simulink model "Exp"  (R2017b)
settings: Solver=FixedStepAuto  StartTime=0.0  StopTime=inf  FixedStep=ts  RelTol=1e-3  EnableMultiTasking=on
values from neighbouring files (symbols this model uses):
  acc_gain = 50    [Init_Exp.m]
  cc = 16    [Init_Exp.m]
  channel = 5    [Init_Exp.m]
  f_gait = 0.1    [Init_Exp.m]
  Kg = 80    [Init_Exp.m]
  R_k = diag([1E-4*[1;1];1E-6*[1;1]])    [Init_Exp.m]
  sigma_p = [0.5 1 100000 100000 100000 100000]'    [Init_Exp.m]
  sigma_pp = [sigma sigma sigma sigma sigma sigma]'    [Init_Exp.m]
  sigma_r = [100000 100000 100000 100000]'    [Init_Exp.m]
  sigma_rr = [sigma sigma sigma sigma]'    [Init_Exp.m]
  systemP = [tau_c2,tau_s2,dqs2,eta2,X2,Y2,J2,tau_c1,tau_s1,dqs1,eta1,X1,Y1,J1]    [Init_Exp.m]
  ts = 0.001    [Init_Exp.m]
  vard = vardtimes*1E-2*[2;1]    [Init_Exp.m]
  vardq = 1E-4*[1;1]    [Init_Exp.m]
  varq = 1E-5*[1;1]    [Init_Exp.m]
undefined symbols (not defined in the file or in its folder): acceleration, command, cxk, desired_acc, desired_position, desired_velocity, DiscIntNeverNeededParam, disturbance, immxk, interaction_force, mkxk, motor_torque, observer, position, velocity, xk
libraries: xpcethercatlib x37, slrtlib x9, simulink x1
(part 2 of 2)

== matlab function Exp/Control/Feedforward&nonlinearFeekbackLinearlization&Observer/disturbance observer ==
  data: TT output; q input; dq input; ddq input; cur input; para input; z input; zz output; d output; c input
function [TT,zz,d] = fcn(q,dq,ddq,cur,para,z,c)


l1=0.42;
tau_c2=para(1);
tau_s2=para(2);
dqs2=para(3);
eta2=para(4);
X2=para(5);
Y2=para(6);
J2=para(7);

tau_c1=para(8);
tau_s1=para(9);
dqs1=para(10);
eta1=para(11);
X1=para(12);
Y1=para(13);
J1=para(14);




%% M matrix
M11=J1+2*l1*(X2*cos(q(2))-Y2*sin(q(2)));
M12=J2+l1*(X2*cos(q(2))-Y2*sin(q(2)));
M21=J2+l1*(X2*cos(q(2))-Y2*sin(q(2)));
M22=J2;

M=[M11,M12;M21,M22];
%% C matrix
C11=-2*l1*(X2*sin(q(2))+Y2*cos(q(2))).*dq(2);
C12=-l1*(X2*sin(q(2))+Y2*cos(q(2))).*dq(2);
C21=l1*(X2*sin(q(2))+Y2*cos(q(2))).*dq(1);
C22=0;

C=[C11,C12;C21,C22];
%% G matrix
G1=9.7925*(X1*sin(q(1))+Y1*cos(q(1)+X2*sin(q(1)+q(2))+Y2*cos(q(1)+q(2))));
G2=9.7925*(X2*sin(q(1)+q(2))+Y2*cos(q(1)+q(2)));

G=[G1;G2];

%% F matrix
F1=(tau_c1+(tau_s1-tau_c1)*exp(-dq(1)/dqs1)).*customSIGN(dq(1))+eta1*dq(1);
F2=(tau_c2+(tau_s2-tau_c2)*exp(-dq(2)/dqs2)).*customSIGN(dq(2))+eta2*dq(2);


F=[F1;F2];

%%

TT=M*ddq+C*dq+G+F;

%% obtain T
% T=cur-F;
T=cur;

%% nonlinear disturbance observer

p=c*[dq(1),dq(1)+dq(2)]';


dt=0.001;
% obtain L matrix
L=c*[1,0;1,1]/M;
zz=(eye(2)-L*dt)*z+L*dt*(C*dq+G-T-p);

d=zz+p;





end



function y=customSIGN(u)
threshold=0.05;
if(u>threshold)
    y=1;
elseif(u<-threshold)
    y=-1;
else
    y=u/threshold;
end


end

== matlab function Exp/Control/Feedforward&nonlinearFeekbackLinearlization&Observer/extended kalman filter ==
  data: xkk output; d output; q input; dq input; ddq input; cur input; para input; D output; xk input; Q_k input; R_k input
function [xkk,d, D] = ExtendedKalmanFilter(q,dq,ddq,cur,para,xk,Q_k,R_k)


persistent   Pk;

if isempty(Pk)
    Pk= 10*eye(6);
end

dt=0.001;
l1=0.42;
tau_c2=para(1);
tau_s2=para(2);
dqs2=para(3);
eta2=para(4);
X2=para(5);
Y2=para(6);
J2=para(7);
tau_c1=para(8);
tau_s1=para(9);
dqs1=para(10);
eta1=para(11);
X1=para(12);
Y1=para(13);
J1=para(14);
%% M matrix
M11=J1+2*l1*(X2*cos(q(2))-Y2*sin(q(2)));
M12=J2+l1*(X2*cos(q(2))-Y2*sin(q(2)));
M21=J2+l1*(X2*cos(q(2))-Y2*sin(q(2)));
M22=J2;
M=[M11,M12;M21,M22];
%% C matrix
C11=-2*l1*(X2*sin(q(2))+Y2*cos(q(2))).*dq(2);
C12=-l1*(X2*sin(q(2))+Y2*cos(q(2))).*dq(2);
C21=l1*(X2*sin(q(2))+Y2*cos(q(2))).*dq(1);
C22=0;
C=[C11,C12;C21,C22];
%% G matrix
G1=9.7925*(X1*sin(q(1))+Y1*cos(q(1)+X2*sin(q(1)+q(2))+Y2*cos(q(1)+q(2))));
G2=9.7925*(X2*sin(q(1)+q(2))+Y2*cos(q(1)+q(2)));
G=[G1;G2];
%% F matrix：fraction
F1=(tau_c1+(tau_s1-tau_c1)*exp(-dq(1)/dqs1)).*customSIGN(dq(1))+eta1*dq(1);
F2=(tau_c2+(tau_s2-tau_c2)*exp(-dq(2)/dqs2)).*customSIGN(dq(2))+eta2*dq(2);
F=[F1;F2];
F=[0;0];
%% native disturbance
D= -cur + (M*ddq+C*dq+G+F);

%% Extended Kalman filter
    H_k = [ 0,0,1,0,0,0;0,0,0,1,0,0;0,0,0,0,1,0;0,0,0,0,0,1];

    y_k = [dq(1),dq(2),q(1),q(2)]';
    % obtain fx
    xdotk=getfxk_1(xk, cur,M,C,G, F);
    xk_=xk + xdotk *dt ;
    
    % obtain F_k
    F_k = GetJacobian_1(xk , cur, F,para);
    
    Pk_=F_k * Pk *  F_k' + Q_k ;
    
    K_k = Pk_ * H_k' /(H_k * Pk_ * H_k' + R_k); 
    
    % Pk = (eye(6)- K_k * H_k)*Pk_;
    Pk = (eye(6)- K_k * H_k)*Pk_*(eye(6)- K_k * H_k)'+ K_k* R_k*K_k';
    
    xkk= xk_ + K_k*(y_k - H_k*xk_);
    
    d =[xkk(1),xkk(2)]';
    
end

function xdot=getfxk_1(x, T, M, C, G, F)

% x= [d dq q]
d=x(1:2);
dq=x(3:4);
q=x(5:6);
invM=inv(M);

xdot=zeros(6,1);
xdot(1:2)=zeros(2,1);
xdot(3:4)=invM*(T+d-C*dq-G-F);

xdot(5:6)=dq;

end

function F_k = GetJacobian_1(x, T, F, para)


dt=0.001;
l1=0.42;
g=9.7925;
X2=para(5);
Y2=para(6);
J2=para(7);
X1=para(12);
Y1=para(13);
J1=para(14);

d=x(1:2);
dq=x(3:4);
q=x(5:6);
%% M matrix
M11=J1+2*l1*(X2*cos(q(2))-Y2*sin(q(2)));
M12=J2+l1*(X2*cos(q(2))-Y2*sin(q(2)));
M21=J2+l1*(X2*cos(q(2))-Y2*sin(q(2)));
M22=J2;
M=[M11,M12;M21,M22];
%% C matrix
C11=-2*l1*(X2*sin(q(2))+Y2*cos(q(2))).*dq(2);
C12=-l1*(X2*sin(q(2))+Y2*cos(q(2))).*dq(2);
C21=l1*(X2*sin(q(2))+Y2*cos(q(2))).*dq(1);
C22=0;
C=[C11,C12;C21,C22];
%% G matrix
G1=g*(X1*sin(q(1))+Y1*cos(q(1)+X2*sin(q(1)+q(2))+Y2*cos(q(1)+q(2))));
G2=g*(X2*sin(q(1)+q(2))+Y2*cos(q(1)+q(2)));
G=[G1;G2];
invM=inv(M);
% calculate xdot
xdot=zeros(6,1);
xdot(1:2)=zeros(2,1);
xdot(3:4)=invM*(T+d-C*dq-G-F);
xdot(5:6)=dq;

f_xk =  xdot;
%%  obtain the numerical Jacobian matrix
gra = zeros(6,6);
for i=1:6
scale = 1E-6;
delta=zeros(6,1);
delta(i)=scale;
%% calculate x_del
x_del=x + delta;
d_del=x_del(1:2);
dq_del=x_del(3:4);
q_del=x_del(5:6);
%% M matrix
M11=J1+2*l1*(X2*cos(q_del(2))-Y2*sin(q_del(2)));
M12=J2+l1*(X2*cos(q_del(2))-Y2*sin(q_del(2)));
M21=J2+l1*(X2*cos(q_del(2))-Y2*sin(q_del(2)));
M22=J2;
M_del=[M11,M12;M21,M22];
%% C matrix
C11=-2*l1*(X2*sin(q_del(2))+Y2*cos(q_del(2))).*dq_del(2);
C12=-l1*(X2*sin(q_del(2))+Y2*cos(q_del(2))).*dq_del(2);
C21=l1*(X2*sin(q_del(2))+Y2*cos(q_del(2))).*dq_del(1);
C22=0;
C_del=[C11,C12;C21,C22];
%% G matrix
G1=g*(X1*sin(q_del(1))+Y1*cos(q_del(1)+X2*sin(q_del(1)+q_del(2))+Y2*cos(q_del(1)+q_del(2))));
G2=g*(X2*sin(q_del(1)+q_del(2))+Y2*cos(q_del(1)+q_del(2)));
G_del=[G1;G2];
invM_del=inv(M_del);
% calculate xdot_del
xdot_del=zeros(6,1);
xdot_del(1:2)=zeros(2,1);
xdot_del(3:4)=invM_del*(T+d_del-C_del*dq_del-G_del-F);
xdot_del(5:6)=dq_del;

f_xk_del= xdot_del ;

J_delta=(f_xk_del - f_xk)*dt;
gra(i,:)=J_delta/scale;

end

F_k = gra'+ eye(6);

end

function y=customSIGN(u)
threshold=0.05;
if(u>threshold)
    y=1;
elseif(u<-threshold)
    y=-1;
else
    y=u/threshold;
end

end

== matlab function Exp/Emergency/MATLAB Function ==
  data: position input; y output; force input
function y = fcn(position, force)

y=0;

if position(1)>0.25*2*pi||position(1)<-0.25*2*pi...
        ||position(2)>0.25*2*pi||position(2)<-0.28*2*pi...
        ||position(3)>0.25*2*pi||position(3)<-0.25*2*pi...
        ||position(4)>0.25*2*pi||position(4)<-0.28*2*pi
    y=1;
else
    y=y;
end

== matlab function Exp/Control/Feedforward&nonlinearFeekbackLinearlization&Observer/MKEKF ==
  data: xkk output; d output; q input; dq input; ddq input; cur input; para input; D output; xk input; num output; Q_k input; Q_maxk input; R_k input; sigma_p input; sigma_r input; XE output; Pk1 output; vec_recp output
function [xkk,d, D,num,XE,Pk1,vec_recp] = MltiKernelExtendedKalmanFilter(q,dq,ddq,cur,para,xk,Q_k,Q_maxk,R_k,sigma_p,sigma_r)


persistent  Pk;

if isempty(Pk)
    Pk= 0.001*eye(6);
end

dt=0.001;
l1=0.42;
tau_c2=para(1);
tau_s2=para(2);
dqs2=para(3);
eta2=para(4);
X2=para(5);
Y2=para(6);
J2=para(7);
tau_c1=para(8);
tau_s1=para(9);
dqs1=para(10);
eta1=para(11);
X1=para(12);
Y1=para(13);
J1=para(14);
%% M matrix
M11=J1+2*l1*(X2*cos(q(2))-Y2*sin(q(2)));
M12=J2+l1*(X2*cos(q(2))-Y2*sin(q(2)));
M21=J2+l1*(X2*cos(q(2))-Y2*sin(q(2)));
M22=J2;
M=[M11,M12;M21,M22];
%% C matrix
C11=-2*l1*(X2*sin(q(2))+Y2*cos(q(2))).*dq(2);
C12=-l1*(X2*sin(q(2))+Y2*cos(q(2))).*dq(2);
C21=l1*(X2*sin(q(2))+Y2*cos(q(2))).*dq(1);
C22=0;
C=[C11,C12;C21,C22];
%% G matrix
G1=9.7925*(X1*sin(q(1))+Y1*cos(q(1)+X2*sin(q(1)+q(2))+Y2*cos(q(1)+q(2))));
G2=9.7925*(X2*sin(q(1)+q(2))+Y2*cos(q(1)+q(2)));
G=[G1;G2];
%% F matrix
F1=(tau_c1+(tau_s1-tau_c1)*exp(-dq(1)/dqs1)).*customSIGN(dq(1))+eta1*dq(1);
F2=(tau_c2+(tau_s2-tau_c2)*exp(-dq(2)/dqs2)).*customSIGN(dq(2))+eta2*dq(2);
F=[F1;F2];
F=[0;0];
%% native disturbance
D= -cur + (M*ddq+C*dq+G+F);

%% Extended Kalman filter
%     sigma_p=[0.5 2 100000 100000 100000 100000]';
%     sigma_r=[100000 100000 100000 100000]';
    H_k = [ 0,0,1,0,0,0;0,0,0,1,0,0;0,0,0,0,1,0;0,0,0,0,0,1];

    y_k = [dq(1),dq(2),q(1),q(2)]';
    % obtain fx
    xdotk=getfxk_1(xk, cur,M,C,G, F);
    xk_=xk + xdotk *dt ;
    
    % obtain F_k
    F_k = GetJacobian_1(xk , cur, F,para);
    
   Pk_=F_k * Pk *  F_k' + Q_k ;   
   %% 
   Pk_max=F_k * Pk *  F_k' + Q_maxk;
   vec_amp=diag(Pk_max)./diag(Pk_);
   vec_recp=1./vec_amp;
   %% %% mkekf
    num=3;
    cnt=num;
    X_t=zeros(6,1);
    K_1=zeros(6,4);
    P_1=zeros(6,6);
    R_1=zeros(4,4);
    XE=zeros(cnt,1);
    %bp = chol(Pk_,'lower') ;
    %Pk_p1=diag(diag(Pk_));
    %Pk_p2=Pk_-Pk_p1;
    bp = chol(Pk_,'lower') ;
    %bp = chol(Pk_p1,'lower') ;
    br = chol(R_k,'lower') ;
    while(num>0) 
    dp= bp\xk_;
    dr= br\y_k;
        % 
    if(num==cnt)
      X_tlast=xk_; 
    else  
      X_tlast=X_t; 
    end
    wp= bp\X_tlast;
    wr= (br)\H_k*X_tlast;
    ep=dp-wp;
    er=dr-wr;
    %  P_ and R
    Cx_array=exp(-ep.*ep./(2*sigma_p.*sigma_p));
    Cy_array=exp(-er.*er./(2*sigma_r.*sigma_r));
    for kk=1:6
        if(Cx_array(kk)<vec_recp(kk))
            Cx_array(kk)=vec_recp(kk);
            num=1;
        end
    end
    
    
    Cx=diag(Cx_array);
    Cy=diag(Cy_array);
        
    R_1=br/Cy*br';
    P_1=bp/Cx*bp';
    %P_1=bp/Cx*bp'+Pk_p2;
    K_1=P_1*H_k'/(H_k*P_1*H_k'+R_1);  
    X_t=xk_+K_1*(y_k-H_k*xk_); 
    
    num=num-1;    
    xe=norm(X_t-X_tlast)/(norm(X_tlast)+0.00001);
    XE(cnt-num)=xe;
    if(xe<0.005)
        break
    end
    
    end 
    %%%%
   
    Pk = (eye(6)- K_1 * H_k)*P_1*(eye(6)- K_1 * H_k)'+ K_1* R_1*K_1';
        
    xkk= X_t;
    
    d =[xkk(1),xkk(2)]';
    
    Pk1=diag(Pk);
end

function xdot=getfxk_1(x, T, M, C, G, F)

% x= [d dq q]
d=x(1:2);
dq=x(3:4);
q=x(5:6);
invM=inv(M);

xdot=zeros(6,1);
xdot(1:2)=zeros(2,1);
xdot(3:4)=invM*(T+d-C*dq-G-F);
xdot(5:6)=dq;

end
function F_k = GetJacobian_1(x, T, F, para)


dt=0.001;
l1=0.42;
g=9.7925;
X2=para(5);
Y2=para(6);
J2=para(7);
X1=para(12);
Y1=para(13);
J1=para(14);

d=x(1:2);
dq=x(3:4);
q=x(5:6);
%% M matrix
M11=J1+2*l1*(X2*cos(q(2))-Y2*sin(q(2)));
M12=J2+l1*(X2*cos(q(2))-Y2*sin(q(2)));
M21=J2+l1*(X2*cos(q(2))-Y2*sin(q(2)));
M22=J2;
M=[M11,M12;M21,M22];
%% C matrix
C11=-2*l1*(X2*sin(q(2))+Y2*cos(q(2))).*dq(2);
C12=-l1*(X2*sin(q(2))+Y2*cos(q(2))).*dq(2);
C21=l1*(X2*sin(q(2))+Y2*cos(q(2))).*dq(1);
C22=0;
C=[C11,C12;C21,C22];
%% G matrix
G1=g*(X1*sin(q(1))+Y1*cos(q(1)+X2*sin(q(1)+q(2))+Y2*cos(q(1)+q(2))));
G2=g*(X2*sin(q(1)+q(2))+Y2*cos(q(1)+q(2)));
G=[G1;G2];
invM=inv(M);
% calculate xdot
xdot=zeros(6,1);
xdot(1:2)=zeros(2,1);
xdot(3:4)=invM*(T+d-C*dq-G-F);
xdot(5:6)=dq;

f_xk =  xdot;
%%  obtain the numerical Jacobian matrix
gra = zeros(6,6);
for i=1:6
scale = 1E-4;
delta=zeros(6,1);
delta(i)=scale;
%% calculate x_del
x_del=x + delta;
d_del=x_del(1:2);
dq_del=x_del(3:4);
q_del=x_del(5:6);
%% M matrix
M11=J1+2*l1*(X2*cos(q_del(2))-Y2*sin(q_del(2)));
M12=J2+l1*(X2*cos(q_del(2))-Y2*sin(q_del(2)));
M21=J2+l1*(X2*cos(q_del(2))-Y2*sin(q_del(2)));
M22=J2;
M_del=[M11,M12;M21,M22];
%% C matrix
C11=-2*l1*(X2*sin(q_del(2))+Y2*cos(q_del(2))).*dq_del(2);
C12=-l1*(X2*sin(q_del(2))+Y2*cos(q_del(2))).*dq_del(2);
C21=l1*(X2*sin(q_del(2))+Y2*cos(q_del(2))).*dq_del(1);
C22=0;
C_del=[C11,C12;C21,C22];
%% G matrix
G1=g*(X1*sin(q_del(1))+Y1*cos(q_del(1)+X2*sin(q_del(1)+q_del(2))+Y2*cos(q_del(1)+q_del(2))));
G2=g*(X2*sin(q_del(1)+q_del(2))+Y2*cos(q_del(1)+q_del(2)));
G_del=[G1;G2];
invM_del=inv(M_del);
% calculate xdot_del
xdot_del=zeros(6,1);
xdot_del(1:2)=zeros(2,1);
xdot_del(3:4)=invM_del*(T+d_del-C_del*dq_del-G_del-F);
xdot_del(5:6)=dq_del;

f_xk_del= xdot_del ;

J_delta=(f_xk_del - f_xk)*dt;
gra(i,:)=J_delta/scale;

end

F_k = gra'+ eye(6);

end

function y=customSIGN(u)
threshold=0.05;
if(u>threshold)
    y=1;
elseif(u<-threshold)
    y=-1;
else
    y=u/threshold;
end

end

== matlab function Exp/6 Axis Force//Torque Sensor/MATLAB Function ==
  data: time input; Bias input; y input; y output; Bias output
function [y, Bias] = fcn(time, Bias, y)

if time <= 3 
    Bias=y;
    y=y*0;
else
    y=y-Bias;
end

end

== matlab function Exp/Control/Feedforward&nonlinearFeekbackLinearlization&Observer/process  ==
  data: vard input; Q_k output; vardq input; varq input
function Q_k = fcn(vard,vardq,varq)

Q_k= diag([vard;vardq;varq]);

== matlab function Exp/Control/Feedforward&nonlinearFeekbackLinearlization&Observer/process 1 ==
  data: vard input; Q_k output; vardq input; varq input; Q_maxk output
function [Q_k,Q_maxk] = fcn(vard,vardq,varq)

Q_k= diag([vard;vardq;varq]);

vardmax=20*1E-2*[2;1];
Q_maxk= diag([vardmax;vardq;varq]);

== matlab function Exp/Control/PD controller/MATLAB Function ==
  data: vele input; y output
function y = fcn(vele)

persistent  veleArr;

if isempty(veleArr)
    veleArr= zeros(20,2);
end

veleArr=circshift(veleArr,1);
veleArr(1,:)=vele;
y1 = var(veleArr(:,1));
y2 = var(veleArr(:,2));
y=[y1;y2];

== matlab function Exp/Emergency/MATLAB Function1 ==
  data: velvar input; y output
function y = fcn(velvar)

if(velvar(1)>0.04||velvar(2)>0.04)
    y=1;
else
    y=0;
end

end

== matlab function Exp/Emergency/MATLAB Function2 ==
  data: cmd input; y output
function y = fcn(cmd)

if(cmd(3)>80||cmd(4)>80)
    y=1;
else
    y=0;
end

end

== matlab function Exp/Control/Feedforward&nonlinearFeekbackLinearlization&Observer/extended kalman filter1 ==
  data: xkk output; xkk1 output; xkk2 output; d output; q input; dq input; cur input; para input; GAMMA output; Qk1 input; Qk2 input; Rk input; T input; mu output; Pkdiag output
function [xkk,xkk1,xkk2,d, GAMMA,mu,Pkdiag] = ExtendedKalmanFilterIMM(q,dq,cur,para,Qk1,Qk2,Rk,T)


persistent  Pk1 Pk2 x1 x2 mu1 mu2

if isempty(Pk1)
    Pk1= 1*eye(6);
end
if isempty(Pk2)
    Pk2= 1*eye(6);
end
if isempty(x1)
    x1= zeros(6,1)+0.01*ones(6,1);
end
if isempty(x2)
    x2= zeros(6,1);
end
if isempty(mu1)
    mu1= 0.5;
end
if isempty(mu2)
    mu2= 0.5;
end

dt=0.001;
l1=0.42;
tau_c2=para(1);
tau_s2=para(2);
dqs2=para(3);
eta2=para(4);
X2=para(5);
Y2=para(6);
J2=para(7);
tau_c1=para(8);
tau_s1=para(9);
dqs1=para(10);
eta1=para(11);
X1=para(12);
Y1=para(13);
J1=para(14);
%% M matrix
M11=J1+2*l1*(X2*cos(q(2))-Y2*sin(q(2)));
M12=J2+l1*(X2*cos(q(2))-Y2*sin(q(2)));
M21=J2+l1*(X2*cos(q(2))-Y2*sin(q(2)));
M22=J2;
M=[M11,M12;M21,M22];
%% C matrix
C11=-2*l1*(X2*sin(q(2))+Y2*cos(q(2))).*dq(2);
C12=-l1*(X2*sin(q(2))+Y2*cos(q(2))).*dq(2);
C21=l1*(X2*sin(q(2))+Y2*cos(q(2))).*dq(1);
C22=0;
C=[C11,C12;C21,C22];
%% G matrix
G1=9.7925*(X1*sin(q(1))+Y1*cos(q(1)+X2*sin(q(1)+q(2))+Y2*cos(q(1)+q(2))));
G2=9.7925*(X2*sin(q(1)+q(2))+Y2*cos(q(1)+q(2)));
G=[G1;G2];
%% F matrix：fraction
F1=(tau_c1+(tau_s1-tau_c1)*exp(-dq(1)/dqs1)).*customSIGN(dq(1))+eta1*dq(1);
F2=(tau_c2+(tau_s2-tau_c2)*exp(-dq(2)/dqs2)).*customSIGN(dq(2))+eta2*dq(2);
F=[F1;F2];
F=[0;0];
%% native disturbance
% D= -cur + (M*ddq+C*dq+G+F);
%% Extended Kalman filter IMM
    H_k = [ 0,0,1,0,0,0;0,0,0,1,0,0;0,0,0,0,1,0;0,0,0,0,0,1];
    y_k = [dq(1),dq(2),q(1),q(2)]';
    % 1: input interaction: c=[mu1 mu2]*T
    c1=T(1,1)*mu1+T(2,1)*mu2;
    c2=T(1,2)*mu1+T(2,2)*mu2;
    % mumu=diag([mu1,mu1])*T   mu=mumu./sum(mumu); % colum normalize
    mu11=T(1,1)*mu1/c1;
    mu12=T(1,2)*mu1/c2;
    mu21=T(2,1)*mu2/c1;
    mu22=T(2,2)*mu2/c2;
    % 2: calculate the initial fusion state vector of model m
    x_pre1=x1*mu11+x2*mu21;
    x_pre2=x1*mu12+x2*mu22;
    % 3: calculate the mixed covariance
    P_pre1=mu11*(Pk1+(x1-x_pre1)*(x1-x_pre1)')+mu21*(Pk2+(x2-x_pre1)*(x2-x_pre1)');
    P_pre2=mu12*(Pk1+(x1-x_pre2)*(x1-x_pre2)')+mu22*(Pk2+(x2-x_pre2)*(x2-x_pre2)');
    % 4: the kalman filter
    % obtain fx
    xdotk1=getfxk_1(x1, cur,M,C,G, F); %xdotk1=getfxk_1(x_pre1, cur,M,C,G, F);
    %xk_=xk + xdotk *dt ;
    % obtain F_k
    F_k1 = GetJacobian_1(x1 , cur, F,para);
    % update 1 
    x1_=x1 + xdotk1 *dt;
    %x1_=F_k1*x_pre1;
    P1_=F_k1*Pk1*F_k1'+Qk1; %P1_=F_k1*P_pre1*F_k1'+Qk1;
    v1=y_k-H_k*x1_;
    S1=H_k*P1_*H_k'+Rk;
    K1=P1_*H_k'/S1;
    x1= x1_+  K1 *v1; % posteriori
    % update 2
    xdotk2=getfxk_1(x2, cur,M,C,G,F); %xdotk2=getfxk_1(x_pre2, cur,M,C,G, F);
    %xk_=xk + xdotk *dt ;
    % obtain F_k
    F_k2 = GetJacobian_1(x2 , cur, F,para);
    x2_=x2 + xdotk2 *dt;
    %x2_=F_k2*x_pre2;
    P2_=F_k2*Pk2*F_k2'+Qk2;%P2_=F_k2*P_pre2*F_k2'+Qk2;
    v2=y_k-H_k*x2_;
    S2=H_k*P2_*H_k'+Rk;
    K2=P2_*H_k'/S2;
    x2= x2_+ K2*v2; % posteriori
    
    % 5: observe the likelihood
    Gamma1=1/sqrt(2*pi*det(S1))*exp(-0.5*v1'*inv(S1)*v1);
    Gamma2=1/sqrt(2*pi*det(S2))*exp(-0.5*v2'*inv(S2)*v2);
    % 6: calculate the filtering covariance matrix
    Pk1=(eye(6)-K1*H_k)*P1_*(eye(6)-K1*H_k)'+K1*Rk*K1';
    Pk2=(eye(6)-K2*H_k)*P2_*(eye(6)-K2*H_k)'+K2*Rk*K2';
    % 7: update the model probability
    c= Gamma1*c1+Gamma2*c2;
    mu1= Gamma1*c1/c;
    mu2= Gamma2*c2/c;
    % 8: output interaction
    xk=mu1*x1+mu2*x2;
    % 9: interact the error covariance matrix
    Pk=mu1*(Pk1+(x1-xk)*(x1-xk)')+mu2*(Pk2+(x2-xk)*(x2-xk)');

    mu=[mu1;mu2];
    xkk=xk;
    xkk1= x1;
    xkk2= x2;
    d =[xkk(1),xkk(2)]';
    Pkdiag=[v1;v2];
    GAMMA=[Gamma1;Gamma2];
end

function xdot=getfxk_1(x, T, M, C, G, F)

% x= [d dq q]
d=x(1:2);
dq=x(3:4);
q=x(5:6);
invM=inv(M);

xdot=zeros(6,1);
xdot(1:2)=zeros(2,1);
xdot(3:4)=invM*(T+d-C*dq-G-F);

xdot(5:6)=dq;

end

function F_k = GetJacobian_1(x, T, F, para)

dt=0.001;
l1=0.42;
g=9.7925;
X2=para(5);
Y2=para(6);
J2=para(7);
X1=para(12);
Y1=para(13);
J1=para(14);

d=x(1:2);
dq=x(3:4);
q=x(5:6);
%% M matrix
M11=J1+2*l1*(X2*cos(q(2))-Y2*sin(q(2)));
M12=J2+l1*(X2*cos(q(2))-Y2*sin(q(2)));
M21=J2+l1*(X2*cos(q(2))-Y2*sin(q(2)));
M22=J2;
M=[M11,M12;M21,M22];
%% C matrix
C11=-2*l1*(X2*sin(q(2))+Y2*cos(q(2))).*dq(2);
C12=-l1*(X2*sin(q(2))+Y2*cos(q(2))).*dq(2);
C21=l1*(X2*sin(q(2))+Y2*cos(q(2))).*dq(1);
C22=0;
C=[C11,C12;C21,C22];
%% G matrix
G1=g*(X1*sin(q(1))+Y1*cos(q(1)+X2*sin(q(1)+q(2))+Y2*cos(q(1)+q(2))));
G2=g*(X2*sin(q(1)+q(2))+Y2*cos(q(1)+q(2)));
G=[G1;G2];
invM=inv(M);
% calculate xdot
xdot=zeros(6,1);
xdot(1:2)=zeros(2,1);
xdot(3:4)=invM*(T+d-C*dq-G-F);
xdot(5:6)=dq;
f_xk =  xdot;
%%  obtain the numerical Jacobian matrix
gra = zeros(6,6);
for i=1:6
scale = 1E-6;
delta=zeros(6,1);
delta(i)=scale;
%% calculate x_del
x_del=x + delta;
d_del=x_del(1:2);
dq_del=x_del(3:4);
q_del=x_del(5:6);
%% M matrix
M11=J1+2*l1*(X2*cos(q_del(2))-Y2*sin(q_del(2)));
M12=J2+l1*(X2*cos(q_del(2))-Y2*sin(q_del(2)));
M21=J2+l1*(X2*cos(q_del(2))-Y2*sin(q_del(2)));
M22=J2;
M_del=[M11,M12;M21,M22];
%% C matrix
C11=-2*l1*(X2*sin(q_del(2))+Y2*cos(q_del(2))).*dq_del(2);
C12=-l1*(X2*sin(q_del(2))+Y2*cos(q_del(2))).*dq_del(2);
C21=l1*(X2*sin(q_del(2))+Y2*cos(q_del(2))).*dq_del(1);
C22=0;
C_del=[C11,C12;C21,C22];
%% G matrix
G1=g*(X1*sin(q_del(1))+Y1*cos(q_del(1)+X2*sin(q_del(1)+q_del(2))+Y2*cos(q_del(1)+q_del(2))));
G2=g*(X2*sin(q_del(1)+q_del(2))+Y2*cos(q_del(1)+q_del(2)));
G_del=[G1;G2];
invM_del=inv(M_del);
% calculate xdot_del
xdot_del=zeros(6,1);
xdot_del(1:2)=zeros(2,1);
xdot_del(3:4)=invM_del*(T+d_del-C_del*dq_del-G_del-F);
xdot_del(5:6)=dq_del;
f_xk_del= xdot_del ;
J_delta=(f_xk_del - f_xk)*dt;
gra(i,:)=J_delta/scale;

end

F_k = gra'+ eye(6);

end

function y=customSIGN(u)
threshold=0.05;
if(u>threshold)
    y=1;
elseif(u<-threshold)
    y=-1;
else
    y=u/threshold;
end

end

== matlab function Exp/Control/Feedforward&nonlinearFeekbackLinearlization&Observer/process 2 ==
  data: vard1 input; vard2 input; vardq input; varq input; Q_k1 output; Q_k2 output
function [Q_k1,Q_k2] = fcn(vard1,vard2,vardq,varq)

Q_k1= diag([vard1;vardq;varq]);
Q_k2= diag([vard2;vardq;varq]);

== matlab function Exp/Control/Gait Generator/Gait Generator ==
  data: t input; gait output; f input; dgait output; ddgait output
function [gait,dgait,ddgait] = fcn(t, f)


A=[19.9072,23.8858,19.9072,23.8858];
B=[7.7114,-23.3998,7.7114,-23.3998];
c=[-0.0781,-1.9451,3.0635,1.1965];
d1=[0.2762,-0.5417,0.2762,-0.5417];
d2=[0.06517,-0.1381,0.06517,-0.1381];
e1=[-0.1455,-1.353,-0.1455,-1.353];
e2=[-0.7061,-0.3798,-0.7061,-0.3798];


q00=[0,0,0,0];
v00=[0,0,0,0];
a00=[0,0,0,0];

q11=zeros(1,4);
v11=zeros(1,4);
a11=zeros(1,4);
T=1;
% initial position vel acc
for i=1:4
    time=0;
    q11(i)=B(i)+A(i)*(sin(2*pi*f*time+c(i))+d1(i)*sin(4*pi*f*time+2*c(i)+e1(i))+d2(i)*sin(6*pi*f*time+3*c(i)+e2(i)));
    v11(i)=A(i)*(2*pi*f*cos(2*pi*f*time+c(i))+4*pi*f*d1(i)*cos(4*pi*f*time+2*c(i)+e1(i))+6*pi*f*d2(i)*cos(6*pi*f*time+3*c(i)+e2(i)));
    a11(i)=-A(i)*(2*pi*f*2*pi*f*sin(2*pi*f*time+c(i))+4*pi*f*4*pi*f*d1(i)*sin(4*pi*f*time+2*c(i)+e1(i))+6*pi*f*6*pi*f*d2(i)*sin(6*pi*f*time+3*c(i)+e2(i)));
end
  


gait=zeros(1,4);
dgait=zeros(1,4);
ddgait=zeros(1,4);

if(t<=1&&t>0)
    for j=1:4
    a0=q00(j);
    a1=v00(j);
    a2=a00(j)/2;
    a3=(20*q11(j)-20*q00(j)-(8*v11(j)+12*v00(j))*T-(3*a00(j)-a11(j))*T^2)/(2*T^3);
    a4=(30*q00(j)-30*q11(j)+(14*v11(j)+16*v00(j))*T+(3*a00(j)-2*a11(j))*T^2)/(2*T^4);
    a5=(12*q11(j)-12*q00(j)-(6*v11(j)+6*v00(j))*T-(a00(j)-a11(j))*T^2)/(2*T^5);%计算五次多项式系数 
    ti=t;
    qi=a0+a1*(ti)+a2*(ti).^2+a3*(ti).^3+a4*(ti).^4+a5*(ti).^5;
    vi=a1+2*a2*(ti)+3*a3*(ti).^2+4*a4*(ti).^3+5*a5*(ti).^4;
    ai=2*a2+6*a3*(ti)+12*a4*(ti).^2+20*a5*(ti).^3;
    gait(j)=qi;
    dgait(j)=vi;
    ddgait(j)=ai;
    end
elseif(t>1)
    time=t-1;
    for i=1:4
    gait(i)=B(i)+A(i)*(sin(2*pi*f*time+c(i))+d1(i)*sin(4*pi*f*time+2*c(i)+e1(i))+d2(i)*sin(6*pi*f*time+3*c(i)+e2(i)));
    dgait(i)=A(i)*(2*pi*f*cos(2*pi*f*time+c(i))+4*pi*f*d1(i)*cos(4*pi*f*time+2*c(i)+e1(i))+6*pi*f*d2(i)*cos(6*pi*f*time+3*c(i)+e2(i)));
    ddgait(i)=-A(i)*(2*pi*f*2*pi*f*sin(2*pi*f*time+c(i))+4*pi*f*4*pi*f*d1(i)*sin(4*pi*f*time+2*c(i)+e1(i))+6*pi*f*6*pi*f*d2(i)*sin(6*pi*f*time+3*c(i)+e2(i)));
    end
else
    gait=zeros(1,4);
    dgait=zeros(1,4);
    ddgait=zeros(1,4);
end

gait=gait/180*pi;
dgait=dgait/180*pi;
ddgait=ddgait/180*pi;

== matlab function Exp/Control/Feedforward&nonlinearFeekbackLinearlization&Observer/extended kalman filter2 ==
  data: xkk output; xkk1 output; xkk2 output; d output; q input; dq input; cur input; para input; GAMMA output; Qk1 input; Qk2 input; Rk input; T input; mu output; v1v2 output; PKK1 output; PKK2 output; Qkk1 output; Qkk2 output
function [xkk,xkk1,xkk2,d, GAMMA,mu,v1v2,PKK1,PKK2,Qkk1,Qkk2]  = ExtendedKalmanFilterIMM(q,dq,cur,para,Qk1,Qk2,Rk,T)


persistent  Pk1 Pk2 x1 x2 mu1 mu2

if isempty(Pk1)
    Pk1= 1*eye(6);
end
if isempty(Pk2)
    Pk2= 1*eye(6);
end
if isempty(x1)
    x1= zeros(6,1);
end
if isempty(x2)
    x2= zeros(6,1);
end
if isempty(mu1)
    mu1= 0.5;
end
if isempty(mu2)
    mu2= 0.5;
end

dt=0.001;
l1=0.42;
tau_c2=para(1);
tau_s2=para(2);
dqs2=para(3);
eta2=para(4);
X2=para(5);
Y2=para(6);
J2=para(7);
tau_c1=para(8);
tau_s1=para(9);
dqs1=para(10);
eta1=para(11);
X1=para(12);
Y1=para(13);
J1=para(14);
%% M matrix
M11=J1+2*l1*(X2*cos(q(2))-Y2*sin(q(2)));
M12=J2+l1*(X2*cos(q(2))-Y2*sin(q(2)));
M21=J2+l1*(X2*cos(q(2))-Y2*sin(q(2)));
M22=J2;
M=[M11,M12;M21,M22];
%% C matrix
C11=-2*l1*(X2*sin(q(2))+Y2*cos(q(2))).*dq(2);
C12=-l1*(X2*sin(q(2))+Y2*cos(q(2))).*dq(2);
C21=l1*(X2*sin(q(2))+Y2*cos(q(2))).*dq(1);
C22=0;
C=[C11,C12;C21,C22];
%% G matrix
G1=9.7925*(X1*sin(q(1))+Y1*cos(q(1)+X2*sin(q(1)+q(2))+Y2*cos(q(1)+q(2))));
G2=9.7925*(X2*sin(q(1)+q(2))+Y2*cos(q(1)+q(2)));
G=[G1;G2];
%% F matrix：fraction
F1=(tau_c1+(tau_s1-tau_c1)*exp(-dq(1)/dqs1)).*customSIGN(dq(1))+eta1*dq(1);
F2=(tau_c2+(tau_s2-tau_c2)*exp(-dq(2)/dqs2)).*customSIGN(dq(2))+eta2*dq(2);
F=[F1;F2];
F=[0;0];
%% native disturbance
% D= -cur + (M*ddq+C*dq+G+F);
%% Extended Kalman filter IMM
    H_k = [ 0,0,1,0,0,0;0,0,0,1,0,0;0,0,0,0,1,0;0,0,0,0,0,1];
    y_k = [dq(1),dq(2),q(1),q(2)]';
    % 1: input interaction: c=[mu1 mu2]*T
    c1=T(1,1)*mu1+T(2,1)*mu2;
    c2=T(1,2)*mu1+T(2,2)*mu2;
    % mumu=diag([mu1,mu1])*T   mu=mumu./sum(mumu); % colum normalize
    mu11=T(1,1)*mu1/c1;
    mu12=T(1,2)*mu1/c2;
    mu21=T(2,1)*mu2/c1;
    mu22=T(2,2)*mu2/c2;
    % 2: calculate the initial fusion state vector of model m
    x_pre1=x1*mu11+x2*mu21;
    x_pre2=x1*mu12+x2*mu22;
    % 3: calculate the mixed covariance
    P_pre1=mu11*(Pk1+(x1-x_pre1)*(x1-x_pre1)')+mu21*(Pk2+(x2-x_pre1)*(x2-x_pre1)');
    P_pre2=mu12*(Pk1+(x1-x_pre2)*(x1-x_pre2)')+mu22*(Pk2+(x2-x_pre2)*(x2-x_pre2)');
    % 4: the kalman filter
    % obtain fx
    xdotk1=getfxk_1(x_pre1, cur,M,C,G, F); %xdotk1=getfxk_1(x_pre1, cur,M,C,G, F);
    %xk_=xk + xdotk *dt ;
    % obtain F_k
    F_k1 = GetJacobian_1(x_pre1 , cur, F,para);
    % update 1 
    x1_=x_pre1 + xdotk1 *dt;
    %x1_=F_k1*x_pre1;
    P1_=F_k1*P_pre1*F_k1'+Qk1; %P1_=F_k1*P_pre1*F_k1'+Qk1;
    v1=y_k-H_k*x1_;
    S1=H_k*P1_*H_k'+Rk;
    K1=P1_*H_k'/S1;
    x1= x1_+  K1 *v1; % posteriori
    % update 2
    xdotk2=getfxk_1(x_pre2, cur,M,C,G,F); %xdotk2=getfxk_1(x_pre2, cur,M,C,G, F);
    %xk_=xk + xdotk *dt ;
    % obtain F_k
    F_k2 = GetJacobian_1(x_pre2 , cur, F,para);
    x2_=x_pre2 + xdotk2 *dt;
    %x2_=F_k2*x_pre2;
    P2_=F_k2*P_pre2*F_k2'+Qk2;%P2_=F_k2*P_pre2*F_k2'+Qk2;
    v2=y_k-H_k*x2_;
    S2=H_k*P2_*H_k'+Rk;
    K2=P2_*H_k'/S2;
    x2= x2_+ K2*v2; % posteriori
    
    % 5: observe the likelihood
    Gamma1=1/sqrt(2*pi*det(S1))*exp(-0.5*v1'/(S1)*v1);
    Gamma2=1/sqrt(2*pi*det(S2))*exp(-0.5*v2'/(S2)*v2);
    % 6: calculate the filtering covariance matrix
    Pk1=(eye(6)-K1*H_k)*P1_*(eye(6)-K1*H_k)'+K1*Rk*K1';
    Pk2=(eye(6)-K2*H_k)*P2_*(eye(6)-K2*H_k)'+K2*Rk*K2';
    % 7: update the model probability
    c= Gamma1*c1+Gamma2*c2;
    mu1= Gamma1*c1/c;
    mu2= Gamma2*c2/c;
    % 8: output interaction
    xk=mu1*x1+mu2*x2;
    % 9: interact the error covariance matrix
    % Pk=mu1*(Pk1+(x1-xk)*(x1-xk)')+mu2*(Pk2+(x2-xk)*(x2-xk)');

    mu=[mu1;mu2];
    xkk=xk;
    xkk1= x1;
    xkk2= x2;
    d =[xkk(1),xkk(2)]';
    v1v2=[v1;v2];
    GAMMA=[Gamma1;Gamma2];
    
    PKK1=diag(P1_);
    PKK2=diag(P2_);
    Qkk1=diag(Qk1);
    Qkk2=diag(Qk2);
end

function xdot=getfxk_1(x, T, M, C, G, F)

% x= [d dq q]
d=x(1:2);
dq=x(3:4);
q=x(5:6);
invM=inv(M);

xdot=zeros(6,1);
xdot(1:2)=zeros(2,1);
xdot(3:4)=invM*(T+d-C*dq-G-F);

xdot(5:6)=dq;

end

function F_k = GetJacobian_1(x, T, F, para)

dt=0.001;
l1=0.42;
g=9.7925;
X2=para(5);
Y2=para(6);
J2=para(7);
X1=para(12);
Y1=para(13);
J1=para(14);

d=x(1:2);
dq=x(3:4);
q=x(5:6);
%% M matrix
M11=J1+2*l1*(X2*cos(q(2))-Y2*sin(q(2)));
M12=J2+l1*(X2*cos(q(2))-Y2*sin(q(2)));
M21=J2+l1*(X2*cos(q(2))-Y2*sin(q(2)));
M22=J2;
M=[M11,M12;M21,M22];
%% C matrix
C11=-2*l1*(X2*sin(q(2))+Y2*cos(q(2))).*dq(2);
C12=-l1*(X2*sin(q(2))+Y2*cos(q(2))).*dq(2);
C21=l1*(X2*sin(q(2))+Y2*cos(q(2))).*dq(1);
C22=0;
C=[C11,C12;C21,C22];
%% G matrix
G1=g*(X1*sin(q(1))+Y1*cos(q(1)+X2*sin(q(1)+q(2))+Y2*cos(q(1)+q(2))));
G2=g*(X2*sin(q(1)+q(2))+Y2*cos(q(1)+q(2)));
G=[G1;G2];
invM=inv(M);
% calculate xdot
xdot=zeros(6,1);
xdot(1:2)=zeros(2,1);
xdot(3:4)=invM*(T+d-C*dq-G-F);
xdot(5:6)=dq;
f_xk =  xdot;
%%  obtain the numerical Jacobian matrix
gra = zeros(6,6);
for i=1:6
scale = 1E-6;
delta=zeros(6,1);
delta(i)=scale;
%% calculate x_del
x_del=x + delta;
d_del=x_del(1:2);
dq_del=x_del(3:4);
q_del=x_del(5:6);
%% M matrix
M11=J1+2*l1*(X2*cos(q_del(2))-Y2*sin(q_del(2)));
M12=J2+l1*(X2*cos(q_del(2))-Y2*sin(q_del(2)));
M21=J2+l1*(X2*cos(q_del(2))-Y2*sin(q_del(2)));
M22=J2;
M_del=[M11,M12;M21,M22];
%% C matrix
C11=-2*l1*(X2*sin(q_del(2))+Y2*cos(q_del(2))).*dq_del(2);
C12=-l1*(X2*sin(q_del(2))+Y2*cos(q_del(2))).*dq_del(2);
C21=l1*(X2*sin(q_del(2))+Y2*cos(q_del(2))).*dq_del(1);
C22=0;
C_del=[C11,C12;C21,C22];
%% G matrix
G1=g*(X1*sin(q_del(1))+Y1*cos(q_del(1)+X2*sin(q_del(1)+q_del(2))+Y2*cos(q_del(1)+q_del(2))));
G2=g*(X2*sin(q_del(1)+q_del(2))+Y2*cos(q_del(1)+q_del(2)));
G_del=[G1;G2];
invM_del=inv(M_del);
% calculate xdot_del
xdot_del=zeros(6,1);
xdot_del(1:2)=zeros(2,1);
xdot_del(3:4)=invM_del*(T+d_del-C_del*dq_del-G_del-F);
xdot_del(5:6)=dq_del;
f_xk_del= xdot_del ;
J_delta=(f_xk_del - f_xk)*dt;
gra(i,:)=J_delta/scale;

end

F_k = gra'+ eye(6);

end

function y=customSIGN(u)
threshold=0.05;
if(u>threshold)
    y=1;
elseif(u<-threshold)
    y=-1;
else
    y=u/threshold;
end

end

== matlab function Exp/Control/Feedforward&nonlinearFeekbackLinearlization&Observer/MKEKF1 ==
  data: xkk output; d output; q input; dq input; ddq input; cur input; para input; D output; xk input; num output; Q_k input; R_k input; sigma_p input; sigma_r input; XE output; Pk1 output
function [xkk,d, D,num,XE,Pk1] = MltiKernelExtendedKalmanFilter(q,dq,ddq,cur,para,xk,Q_k,R_k,sigma_p,sigma_r)


persistent  Pk;

if isempty(Pk)
    Pk= 0.001*eye(6);
end

dt=0.001;
l1=0.42;
tau_c2=para(1);
tau_s2=para(2);
dqs2=para(3);
eta2=para(4);
X2=para(5);
Y2=para(6);
J2=para(7);
tau_c1=para(8);
tau_s1=para(9);
dqs1=para(10);
eta1=para(11);
X1=para(12);
Y1=para(13);
J1=para(14);
%% M matrix
M11=J1+2*l1*(X2*cos(q(2))-Y2*sin(q(2)));
M12=J2+l1*(X2*cos(q(2))-Y2*sin(q(2)));
M21=J2+l1*(X2*cos(q(2))-Y2*sin(q(2)));
M22=J2;
M=[M11,M12;M21,M22];
%% C matrix
C11=-2*l1*(X2*sin(q(2))+Y2*cos(q(2))).*dq(2);
C12=-l1*(X2*sin(q(2))+Y2*cos(q(2))).*dq(2);
C21=l1*(X2*sin(q(2))+Y2*cos(q(2))).*dq(1);
C22=0;
C=[C11,C12;C21,C22];
%% G matrix
G1=9.7925*(X1*sin(q(1))+Y1*cos(q(1)+X2*sin(q(1)+q(2))+Y2*cos(q(1)+q(2))));
G2=9.7925*(X2*sin(q(1)+q(2))+Y2*cos(q(1)+q(2)));
G=[G1;G2];
%% F matrix
F1=(tau_c1+(tau_s1-tau_c1)*exp(-dq(1)/dqs1)).*customSIGN(dq(1))+eta1*dq(1);
F2=(tau_c2+(tau_s2-tau_c2)*exp(-dq(2)/dqs2)).*customSIGN(dq(2))+eta2*dq(2);
F=[F1;F2];
F=[0;0];
%% native disturbance
D= -cur + (M*ddq+C*dq+G+F);

%% Extended Kalman filter
%     sigma_p=[0.5 2 100000 100000 100000 100000]';
%     sigma_r=[100000 100000 100000 100000]';
    H_k = [ 0,0,1,0,0,0;0,0,0,1,0,0;0,0,0,0,1,0;0,0,0,0,0,1];

    y_k = [dq(1),dq(2),q(1),q(2)]';
    % obtain fx
    xdotk=getfxk_1(xk, cur,M,C,G, F);
    xk_=xk + xdotk *dt ;
    
    % obtain F_k
    F_k = GetJacobian_1(xk , cur, F,para);
    
    Pk_=F_k * Pk *  F_k' + Q_k ;    
    %%%%
    num=3;
    cnt=num;
    X_t=zeros(6,1);
    K_1=zeros(6,4);
    P_1=zeros(6,6);
    R_1=zeros(4,4);
    XE=zeros(cnt,1);
    %bp = chol(Pk_,'lower') ;
    %Pk_p1=diag(diag(Pk_));
    %Pk_p2=Pk_-Pk_p1;
    bp = chol(Pk_,'lower') ;
    %bp = chol(Pk_p1,'lower') ;
    br = chol(R_k,'lower') ;
    while(num>0) 
    dp= bp\xk_;
    dr= br\y_k;
        % 
    if(num==cnt)
      X_tlast=xk_; 
    else  
      X_tlast=X_t; 
    end
    wp= bp\X_tlast;
    wr= (br)\H_k*X_tlast;
    ep=dp-wp;
    er=dr-wr;
    %  P_ and R
    Cx_array=exp(-ep.*ep./(2*sigma_p.*sigma_p));
    Cy_array=exp(-er.*er./(2*sigma_r.*sigma_r));
    for kk=1:6
        if(Cx_array(kk)<0.2)
            Cx_array(kk)=0.2;
            num=1;
        end
    end
    Cx=diag(Cx_array);
    Cy=diag(Cy_array);
        
    R_1=br/Cy*br';
    P_1=bp/Cx*bp';
    %P_1=bp/Cx*bp'+Pk_p2;
    K_1=P_1*H_k'/(H_k*P_1*H_k'+R_1);  
    X_t=xk_+K_1*(y_k-H_k*xk_); 
    
    num=num-1;    
    xe=norm(X_t-X_tlast)/(norm(X_tlast)+0.00001);
    XE(cnt-num)=xe;
    if(xe<0.005)
        break
    end
    
    end 
    %%%%
   
    Pk = (eye(6)- K_1 * H_k)*P_1*(eye(6)- K_1 * H_k)'+ K_1* R_1*K_1';
        
    xkk= X_t;
    
    d =[xkk(1),xkk(2)]';
    
    Pk1=diag(Pk);
end

function xdot=getfxk_1(x, T, M, C, G, F)

% x= [d dq q]
d=x(1:2);
dq=x(3:4);
q=x(5:6);
invM=inv(M);

xdot=zeros(6,1);
xdot(1:2)=zeros(2,1);
xdot(3:4)=invM*(T+d-C*dq-G-F);
xdot(5:6)=dq;

end
function F_k = GetJacobian_1(x, T, F, para)


dt=0.001;
l1=0.42;
g=9.7925;
X2=para(5);
Y2=para(6);
J2=para(7);
X1=para(12);
Y1=para(13);
J1=para(14);

d=x(1:2);
dq=x(3:4);
q=x(5:6);
%% M matrix
M11=J1+2*l1*(X2*cos(q(2))-Y2*sin(q(2)));
M12=J2+l1*(X2*cos(q(2))-Y2*sin(q(2)));
M21=J2+l1*(X2*cos(q(2))-Y2*sin(q(2)));
M22=J2;
M=[M11,M12;M21,M22];
%% C matrix
C11=-2*l1*(X2*sin(q(2))+Y2*cos(q(2))).*dq(2);
C12=-l1*(X2*sin(q(2))+Y2*cos(q(2))).*dq(2);
C21=l1*(X2*sin(q(2))+Y2*cos(q(2))).*dq(1);
C22=0;
C=[C11,C12;C21,C22];
%% G matrix
G1=g*(X1*sin(q(1))+Y1*cos(q(1)+X2*sin(q(1)+q(2))+Y2*cos(q(1)+q(2))));
G2=g*(X2*sin(q(1)+q(2))+Y2*cos(q(1)+q(2)));
G=[G1;G2];
invM=inv(M);
% calculate xdot
xdot=zeros(6,1);
xdot(1:2)=zeros(2,1);
xdot(3:4)=invM*(T+d-C*dq-G-F);
xdot(5:6)=dq;

f_xk =  xdot;
%%  obtain the numerical Jacobian matrix
gra = zeros(6,6);
for i=1:6
scale = 1E-4;
delta=zeros(6,1);
delta(i)=scale;
%% calculate x_del
x_del=x + delta;
d_del=x_del(1:2);
dq_del=x_del(3:4);
q_del=x_del(5:6);
%% M matrix
M11=J1+2*l1*(X2*cos(q_del(2))-Y2*sin(q_del(2)));
M12=J2+l1*(X2*cos(q_del(2))-Y2*sin(q_del(2)));
M21=J2+l1*(X2*cos(q_del(2))-Y2*sin(q_del(2)));
M22=J2;
M_del=[M11,M12;M21,M22];
%% C matrix
C11=-2*l1*(X2*sin(q_del(2))+Y2*cos(q_del(2))).*dq_del(2);
C12=-l1*(X2*sin(q_del(2))+Y2*cos(q_del(2))).*dq_del(2);
C21=l1*(X2*sin(q_del(2))+Y2*cos(q_del(2))).*dq_del(1);
C22=0;
C_del=[C11,C12;C21,C22];
%% G matrix
G1=g*(X1*sin(q_del(1))+Y1*cos(q_del(1)+X2*sin(q_del(1)+q_del(2))+Y2*cos(q_del(1)+q_del(2))));
G2=g*(X2*sin(q_del(1)+q_del(2))+Y2*cos(q_del(1)+q_del(2)));
G_del=[G1;G2];
invM_del=inv(M_del);
% calculate xdot_del
xdot_del=zeros(6,1);
xdot_del(1:2)=zeros(2,1);
xdot_del(3:4)=invM_del*(T+d_del-C_del*dq_del-G_del-F);
xdot_del(5:6)=dq_del;

f_xk_del= xdot_del ;

J_delta=(f_xk_del - f_xk)*dt;
gra(i,:)=J_delta/scale;

end

F_k = gra'+ eye(6);

end

function y=customSIGN(u)
threshold=0.05;
if(u>threshold)
    y=1;
elseif(u<-threshold)
    y=-1;
else
    y=u/threshold;
end

end

== matlab function Exp/Control/Feedforward&nonlinearFeekbackLinearlization&Observer/process 3 ==
  data: vard input; Q_k output; vardq input; varq input
function Q_k = fcn(vard,vardq,varq)

Q_k= diag([vard;vardq;varq]);

== matlab function Exp/Emergency/MATLAB Function3 ==
  data: time input; y output
function y = fcn(time)

if(time>50)
    y=1;
else
    y=0;
end

end
